simulink model "Elevator_Height_Reset"  (R2023b)
settings: Solver=VariableStepDiscrete  StartTime=0.0  StopTime=22  MaxStep=0.02  RelTol=1e-3
undefined symbols (not defined in the file): Elevator_Height_PickupLower_Reset, Elevator_Height_Top_Reset, Elevator_MotorRev_to_Inch
libraries: simulink x2
settings Model: Creator=Blank  LastModifiedBy=ander

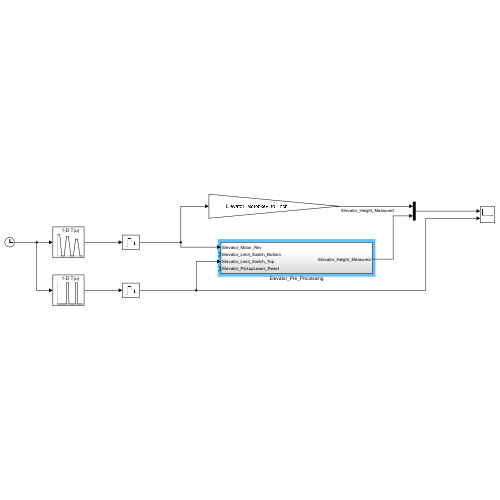
[thumbnail: Simulink's stored preview of the top-level diagram]
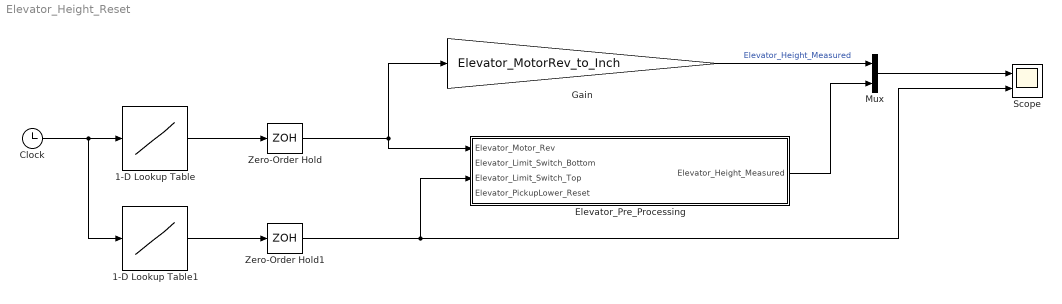
== system Elevator_Height_Reset ==
  1-D Lookup Table : Lookup_n-D  NumberOfTableDimensions=1  BreakpointsForDimension1=[0 2 4 6 8 10 12 14 16 18 20 22]  Table=100-[0 0 100 100 10 10 100 100 20 20 100 100]  InternalRulePriority=Speed  RndMeth=Simplest
  1-D Lookup Table1 : Lookup_n-D  NumberOfTableDimensions=1  BreakpointsForDimension1=[0 2 4 6 7.98 8 10 10.02 12 14 15.98 16 17.98 18 20 22]  Table=[0 0 0 0 0 1 1 0 0 0 0 1 1 0 0 0]  InternalRulePriority=Speed  RndMeth=Simplest
  Clock : Clock
  Elevator_Pre_Processing : Subsystem
  Gain : Gain  Gain=Elevator_MotorRev_to_Inch
  Mux : Mux  Inputs=2
  Scope : Scope  NumInputPorts=2
  Zero-Order Hold : ZeroOrderHold  SampleTime=0.02
  Zero-Order Hold1 : ZeroOrderHold  SampleTime=0.02
  wires:
  Clock/1 -> 1-D Lookup Table1/1, 1-D Lookup Table/1
  1-D Lookup Table/1 -> Zero-Order Hold/1
  Gain/1 -> Mux/1  "Elevator_Height_Measured"
  Mux/1 -> Scope/1
  Elevator_Pre_Processing/1(Elevator_Height_Measured) -> Mux/2
  1-D Lookup Table1/1 -> Zero-Order Hold1/1
  Zero-Order Hold/1 -> Elevator_Pre_Processing/1(Elevator_Motor_Rev), Gain/1
  Zero-Order Hold1/1 -> Elevator_Pre_Processing/3(Elevator_Limit_Switch_Top), Scope/2

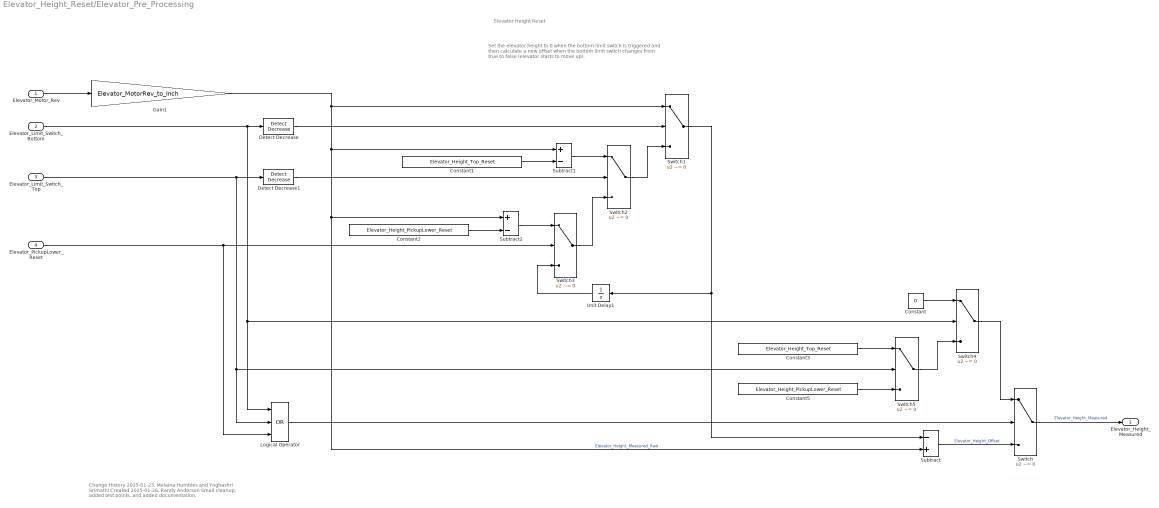
== system Elevator_Height_Reset/Elevator_Pre_Processing ==
  note: Set the elevator height to 0 when the bottom limit switch is triggered
      | and then calculate a new offset when the bottom limit switch changes
      | from true to false (elevator starts to move up).
  note: Elevator Height Reset
  note: Change History
      | 2025-01-23, Melaina Humbles and Yoghashri Srimathi
      | Created
      | 2025-01-26, Randy Anderson
      | Small cleanup, added test points, and added documentation.
  Elevator_Motor_Rev : Inport
  Elevator_Limit_Switch_Bottom : Inport  Port=2
  Elevator_Limit_Switch_Top : Inport  Port=3
  Elevator_PickupLower_Reset : Inport  Port=4
  Constant : Constant  Value=0
  Constant1 : Constant  Value=Elevator_Height_Top_Reset
  Constant2 : Constant  Value=Elevator_Height_PickupLower_Reset
  Constant3 : Constant  Value=Elevator_Height_Top_Reset
  Constant5 : Constant  Value=Elevator_Height_PickupLower_Reset
  Detect Decrease : simulink/Logic and Bit Operations/Detect Decrease  vinit=0.0  OutDataTypeStr=boolean
  Detect Decrease1 : simulink/Logic and Bit Operations/Detect Decrease  vinit=0.0  OutDataTypeStr=boolean
  Gain1 : Gain  Gain=Elevator_MotorRev_to_Inch
  Logical Operator : Logic  Operator=OR  Inputs=3  AllPortsSameDT=off  OutDataTypeStr=boolean
  Subtract : Sum  Inputs=-+
  Subtract1 : Sum  Inputs=+-
  Subtract2 : Sum  Inputs=+-
  Switch{,1..5} (6 alike) : Switch  Criteria=u2 ~= 0  SaturateOnIntegerOverflow=off  InputSameDT=off
  Unit Delay1 : UnitDelay  SampleTime=-1  HasFrameUpgradeWarning=on
  Elevator_Height_Measured : Outport
  wires:
  Elevator_Limit_Switch_Bottom/1 -> Logical Operator/1, Switch4/2, Detect Decrease/1
  Elevator_Motor_Rev/1 -> Gain1/1
  Detect Decrease/1 -> Switch1/2
  Switch1/1 -> Subtract/1, Unit Delay1/1
  Switch/1 -> Elevator_Height_Measured/1  "Elevator_Height_Measured"
  Subtract/1 -> Switch/3  "Elevator_Height_Offset"
  Gain1/1 -> Subtract2/1, Subtract/2, Subtract1/1, Switch1/1  "Elevator_Height_Measured_Raw"
  Switch2/1 -> Switch1/3
  Detect Decrease1/1 -> Switch2/2
  Elevator_Limit_Switch_Top/1 -> Logical Operator/2, Switch5/2, Detect Decrease1/1
  Subtract1/1 -> Switch2/1
  Constant1/1 -> Subtract1/2
  Constant2/1 -> Subtract2/2
  Subtract2/1 -> Switch3/1
  Switch3/1 -> Switch2/3
  Unit Delay1/1 -> Switch3/3
  Constant/1 -> Switch4/1
  Switch5/1 -> Switch4/3
  Constant3/1 -> Switch5/1
  Elevator_PickupLower_Reset/1 -> Logical Operator/3, Switch3/2
  Constant5/1 -> Switch5/3
  Switch4/1 -> Switch/1
  Logical Operator/1 -> Switch/2
